simulink model "Q9_BLDC"  (R2020b)
settings: Solver=VariableStepAuto  StartTime=0.0  StopTime=10.0  RelTol=1e-3
values from neighbouring files (symbols this model uses):
  B = 0.01    [Data_dict.sldd]    (also in Design_Data.m)
  KePhi = 1.6    [Data_dict.sldd]    (also in Design_Data.m)
  Ra = 0.5    [Data_dict.sldd]    (also in Design_Data.m)
  Tau_a = 0.2    [Data_dict.sldd]    (also in Design_Data.m)
  Tau_m = 500.0    [Data_dict.sldd]    (also in Design_Data.m = 500)
  TL = 50.0    [Data_dict.sldd]    (also in Design_Data.m = 50)
  Va = 160.0    [Data_dict.sldd]    (also in Design_Data.m = 200)
settings Model: DataDictionary=Data_dict.sldd  Creator=Shree  LastModifiedBy=Shree

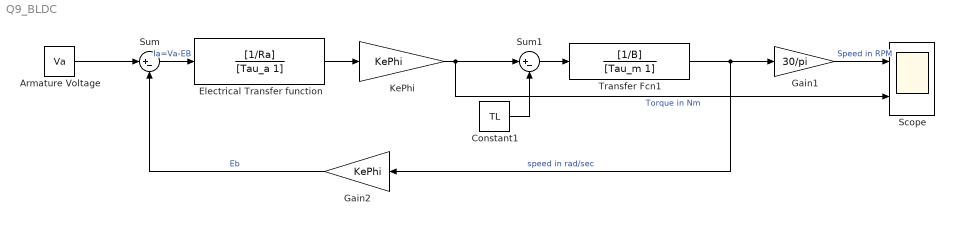
== system Q9_BLDC ==
  Armature Voltage : Constant  Value=Va
  Constant1 : Constant  Value=TL
  Electrical Transfer function : TransferFcn  Numerator=[1/Ra]  Denominator=[Tau_a 1]
  Gain1 : Gain  Gain=30/pi
  Gain2 : Gain  Gain=KePhi
  KePhi : Gain  Gain=KePhi
  Scope : Scope  NumInputPorts=2
  Sum : Sum  Inputs=|+-
  Sum1 : Sum  Inputs=|+-
  Transfer Fcn1 : TransferFcn  Numerator=[1/B]  Denominator=[Tau_m 1]
  wires:
  Sum/1 -> Electrical Transfer function/1  "Ia=Va-EB"
  Electrical Transfer function/1 -> KePhi/1
  KePhi/1 -> Scope/2, Sum1/1  "Torque in Nm"
  Sum1/1 -> Transfer Fcn1/1
  Transfer Fcn1/1 -> Gain1/1, Gain2/1  "speed in rad/sec"
  Gain1/1 -> Scope/1  "Speed in RPM"
  Gain2/1 -> Sum/2  "Eb"
  Armature Voltage/1 -> Sum/1
  Constant1/1 -> Sum1/2
